simulink model "OuterLoop_Control_Harness_HLR_6"  (R2026b)
settings: Solver=FixedStepDiscrete  EnableMultiTasking=on
settings Model: DataDictionary=DD_OuterLoop_Control.sldd  Creator=The MathWorks, Inc.  LastModifiedBy=The MathWorks, Inc.
settings DataIOCC: InputTimeTolerance=off  LimitDataPoints=on
settings OptimizationCC: BlockReduction=off  DefaultParameterBehavior=Inlined  EfficientFloat2IntCast=on  EfficientMapNaN2IntZero=off  EfficientTunableParamExpr=on  EnhancedBackFolding=on  InlineInvariantSignals=on  LifeSpan=inf  MaxStackSize=inf  OptimizeBlockOrder=speed  PassReuseOutputArgsAs=Individual arguments  UseDivisionForNetSlopeComputation=on  UseFloatMulNetSlope=on
settings DebuggingCC: AlgebraicLoopMsg=error  AllowSymbolicDim=off  ArithmeticOperatorsInVariantConditions=warning  ArtificialAlgebraicLoopMsg=error  AssertControl=DisableAll  BlockPriorityViolationMsg=error  BusObjectLabelMismatch=error  CheckMatrixSingularityMsg=error  InheritedTsInSrcMsg=error  IntegerOverflowMsg=error  IntegerSaturationMsg=error  ModelReferenceDataLoggingMessage=error  ModelReferenceIOMismatchMessage=error  ModelReferenceSymbolNameMessage=none  NonBusSignalsTreatedAsBus=error  ParameterPrecisionLossMsg=error  ParameterTunabilityLossMsg=error  ParameterUnderflowMsg=error  PregeneratedLibrarySubsystemCodeDiagnostic=none  ReadBeforeWriteMsg=EnableAllAsError  RootOutportRequireBusObject=error  SFExecutionAtInitializationDiag=none  SFInvalidInputDataAccessInChartInitDiag=error  SFTransitionActionBeforeConditionDiag=error  SFTransitionOutsideNaturalParentDiag=error  SFUndirectedBroadcastEventsDiag=error  SFUnreachableExecutionPathDiag=error  SFcnCompatibilityMsg=error  SaveWithDisabledLinksMsg=error  SaveWithParameterizedLinksMsg=error  SigSpecEnsureSampleTimeMsg=error  SignalInfNanChecking=error  SignalLabelMismatchMsg=error  SignalRangeChecking=error  SingleTaskRateTransMsg=error  SolverPrmCheckMsg=error  StateNameClashWarn=warning  StrictBusMsg=ErrorOnBusTreatedAsVector  TasksWithSamePriorityMsg=error  UnconnectedInputMsg=error  UnconnectedLineMsg=error  UnconnectedOutputMsg=error  UnderSpecifiedDataTypeMsg=error  UniqueDataStoreMsg=error  UnknownTsInhSupMsg=error  UnnecessaryDatatypeConvMsg=warning  VectorMatrixConversionMsg=error  WriteAfterReadMsg=EnableAllAsError  WriteAfterWriteMsg=EnableAllAsError
settings HardwareCC: ProdHWDeviceType=ARM Compatible->ARM 10  ProdLargestAtomicInteger=Long
settings ModelReferenceCC: ModelReferenceNumInstancesAllowed=Single  PropagateSignalLabelsOutOfModel=off
settings SFSimCC: CustomCodeUndefinedFunction=UseInterfaceOnly  EnableRuntimeRecursion=off  MATLABDynamicMemAlloc=off
settings RTWCC: BuildConfiguration=Faster Runs  DLArmComputeVersion=19.05  Description=Embedded Coder  GenCodeOnly=on  GenerateCodeMetricsReport=on  GenerateReport=on  GenerateTraceInfo=on  GenerateTraceReport=on  GenerateTraceReportEml=on  GenerateTraceReportSf=on  GenerateTraceReportSl=on  IncludeHyperlinkInReport=on  LaunchReport=on  SystemTargetFile=ert.tlc  TemplateMakefile=ert_default_tmf
settings CodeAppCC: ForceParamTrailComments=on  IgnoreCustomStorageClasses=off  MATLABFcnDesc=on  ReqsInCode=on  StateflowObjectComments=on
settings ERTTargetCC: CastingMode=Standards  DynamicArrayContainerType=coder::array  EnableSignedLeftShifts=off  EnableSignedRightShifts=off  GenerateSampleERTMain=on  GenerateSharedConstants=off  IncludeMdlTerminateFcn=off  ParenthesesLevel=Maximum  PreserveExpressionOrder=on  PreserveIfCondition=on  RemoveDisableFunc=on  SubcomponentCodeInterfacePackaging=Nonreusable function  SupportAbsoluteTime=off  SupportNonFinite=off  SuppressErrorStatus=on  UtilityFuncGeneration=Shared location

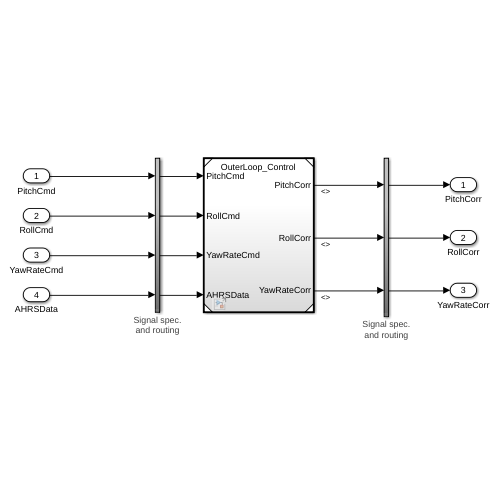
[thumbnail: Simulink's stored preview of the top-level diagram]
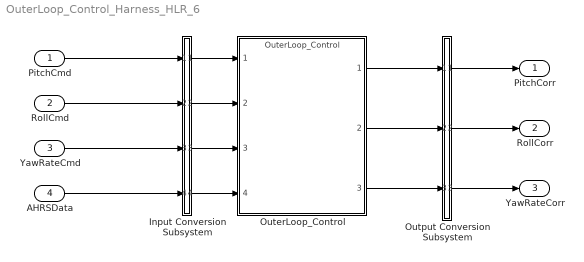
== system OuterLoop_Control_Harness_HLR_6 ==
  PitchCmd : Inport  OutDataTypeStr=double  PortDimensions=[1]  SampleTime=0.01
  RollCmd : Inport  Port=2  OutDataTypeStr=double  PortDimensions=[1]  SampleTime=0.01
  YawRateCmd : Inport  Port=3  OutDataTypeStr=double  PortDimensions=[1]  SampleTime=0.01
  AHRSData : Inport  Port=4  OutDataTypeStr=double  PortDimensions=[5]  SampleTime=0.01
  Input Conversion Subsystem : Subsystem  Tag=__SLT_ICS__  Description=|
      | Signal spec.
      | and routing
      settings: AttributesFormatString=%<Description>
  OuterLoop_Control : ModelReference  ModelNameDialog=OuterLoop_Control  SimulationMode=Normal  ModelReferenceVersion=7.3
  Output Conversion Subsystem : Subsystem  Tag=__SLT_OCS__  Description=|
      | Signal spec.
      | and routing
      settings: AttributesFormatString=%<Description>
  PitchCorr : Outport
  RollCorr : Outport  Port=2
  YawRateCorr : Outport  Port=3
  wires:
  PitchCmd/1 -> Input Conversion Subsystem/1(Inport_1)
  RollCmd/1 -> Input Conversion Subsystem/2(Inport_2)
  YawRateCmd/1 -> Input Conversion Subsystem/3(Inport_3)
  AHRSData/1 -> Input Conversion Subsystem/4(Inport_4)
  Output Conversion Subsystem/1(Outport_1) -> PitchCorr/1
  Output Conversion Subsystem/2(Outport_2) -> RollCorr/1
  Output Conversion Subsystem/3(Outport_3) -> YawRateCorr/1
  Input Conversion Subsystem/1(Outport_1) -> OuterLoop_Control/1
  Input Conversion Subsystem/2(Outport_2) -> OuterLoop_Control/2
  Input Conversion Subsystem/3(Outport_3) -> OuterLoop_Control/3
  Input Conversion Subsystem/4(Outport_4) -> OuterLoop_Control/4
  OuterLoop_Control/1 -> Output Conversion Subsystem/1(Inport_1)
  OuterLoop_Control/2 -> Output Conversion Subsystem/2(Inport_2)
  OuterLoop_Control/3 -> Output Conversion Subsystem/3(Inport_3)

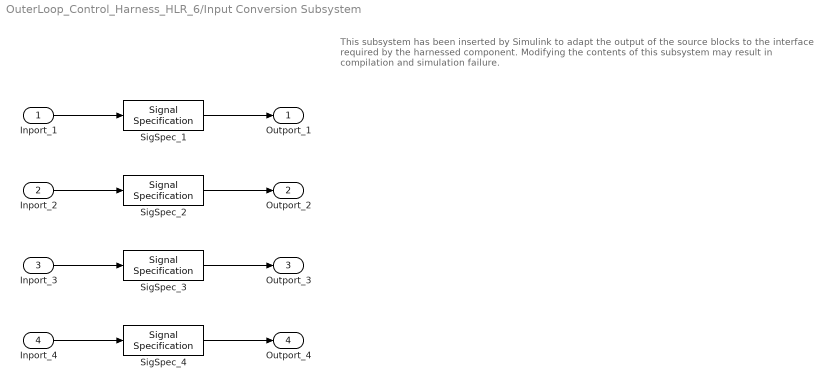
== system OuterLoop_Control_Harness_HLR_6/Input Conversion Subsystem ==
  note: This subsystem has been inserted by Simulink to adapt the output of the source blocks to the interface required by the harnessed component.
      |  Modifying the contents of this subsystem may result in compilation and simulation failure.
  Inport_1 : Inport
  Inport_2 : Inport  Port=2
  Inport_3 : Inport  Port=3
  Inport_4 : Inport  Port=4
  SigSpec_1 : SignalSpecification  OutDataTypeStr=double  Dimensions=[1]  SampleTime=0.01
  SigSpec_2 : SignalSpecification  OutDataTypeStr=double  Dimensions=[1]  SampleTime=0.01
  SigSpec_3 : SignalSpecification  OutDataTypeStr=double  Dimensions=[1]  SampleTime=0.01
  SigSpec_4 : SignalSpecification  OutDataTypeStr=double  Dimensions=[5]  SampleTime=0.01
  Outport_1 : Outport
  Outport_2 : Outport  Port=2
  Outport_3 : Outport  Port=3
  Outport_4 : Outport  Port=4
  wires:
  SigSpec_1/1 -> Outport_1/1
  Inport_1/1 -> SigSpec_1/1
  SigSpec_2/1 -> Outport_2/1
  Inport_2/1 -> SigSpec_2/1
  SigSpec_3/1 -> Outport_3/1
  Inport_3/1 -> SigSpec_3/1
  SigSpec_4/1 -> Outport_4/1
  Inport_4/1 -> SigSpec_4/1

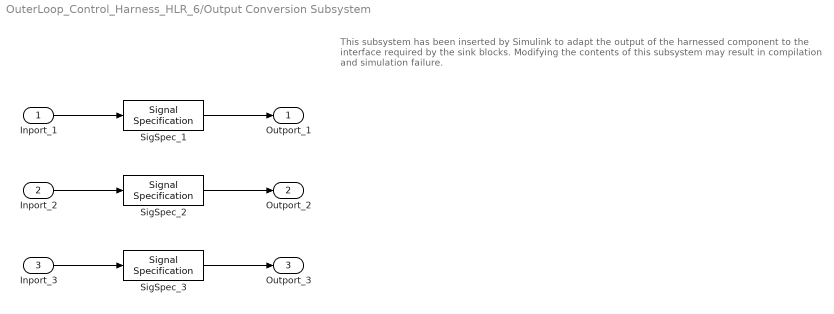
== system OuterLoop_Control_Harness_HLR_6/Output Conversion Subsystem ==
  note: This subsystem has been inserted by Simulink to adapt the output of the harnessed component to the interface required by the sink blocks.
      |  Modifying the contents of this subsystem may result in compilation and simulation failure.
  Inport_1 : Inport
  Inport_2 : Inport  Port=2
  Inport_3 : Inport  Port=3
  SigSpec_1 : SignalSpecification  OutDataTypeStr=double  Dimensions=[1]  SampleTime=0.01
  SigSpec_2 : SignalSpecification  OutDataTypeStr=double  Dimensions=[1]  SampleTime=0.01
  SigSpec_3 : SignalSpecification  OutDataTypeStr=double  Dimensions=[1]  SampleTime=0.01
  Outport_1 : Outport
  Outport_2 : Outport  Port=2
  Outport_3 : Outport  Port=3
  wires:
  Inport_1/1 -> SigSpec_1/1
  SigSpec_1/1 -> Outport_1/1
  Inport_2/1 -> SigSpec_2/1
  SigSpec_2/1 -> Outport_2/1
  Inport_3/1 -> SigSpec_3/1
  SigSpec_3/1 -> Outport_3/1
